simulink model "STOICAL_example_3_Step00_ExistingModell"  (R2014b)
settings: Solver=ode4  StartTime=0.0  StopTime=1  FixedStep=50E-6  RelTol=1e-3
model workspace (MAT data in the model file):
  STOVICAL.SignalSaveOptions.ReturnWorkspaceOutputs = 'on'
  STOVICAL.SignalSaveOptions.ReturnWorkspaceOutputsName = 'simout_obj'
  STOVICAL.SignalSaveOptions.SignalLogging = 'on'
  STOVICAL.SignalSaveOptions.SignalLoggingSaveFormat = 'Dataset'
  STOVICAL.SignalSaveOptions.SignalLoggingName = 'STOVICAL_LoggedSignals'
  STOVICAL.ParameterDefinition.BlkNameFull{1} = 'Step amplitude
    | #PARAM#Amplitude'
  STOVICAL.ParameterDefinition.BlkNameFull{2} = 'Dynamic System
    | #PARAM#w0#damp'
  STOVICAL.ParameterDefinition.BlkNameFull{3} = 'Static System
    | modelled
    | by gain block
    | #PARAM#SystemGain'
  STOVICAL.ParameterDefinition.BlkNameFull{4} = 'Dynamic System
    | #PARAM#w0#damp'
  STOVICAL.ParameterDefinition.BlkNameShort{1} = 'Step amplitude
    | '
  STOVICAL.ParameterDefinition.BlkNameShort{2} = 'Dynamic System
    | '
  STOVICAL.ParameterDefinition.BlkNameShort{3} = 'Static System
    | modelled
    | by gain block
    | '
  STOVICAL.ParameterDefinition.BlkNameShort{4} = 'Dynamic System
    | '
  STOVICAL.ParameterDefinition.BlkHandle = [8.0009765625; 15.0009765625; 21.0024414062; 15.0009765625]
  STOVICAL.ParameterDefinition.ParamName = {'Amplitude'; 'w0'; 'SystemGain'; 'damp'}
  STOVICAL.ParameterDefinition.BlkPath{1} = 'STOICAL_example_2_Step03_Activation/#UNIT#Stimulus/Step amplitude
    | #PARAM#Amplitude'
  STOVICAL.ParameterDefinition.BlkPath{2} = 'STOICAL_example_2_Step03_Activation/#UNIT#System/Dynamic System
    | #PARAM#w0#damp'
  STOVICAL.ParameterDefinition.BlkPath{3} = 'STOICAL_example_2_Step03_Activation/#UNIT#System/Static System
    | modelled
    | by gain block
    | #PARAM#SystemGain'
  STOVICAL.ParameterDefinition.BlkPath{4} = 'STOICAL_example_2_Step03_Activation/#UNIT#System/Dynamic System
    | #PARAM#w0#damp'
  STOVICAL.ParameterDefinition.BlkType = {'Constant'; 'SubSystem'; 'Gain'; 'SubSystem'}
  STOVICAL.ParameterDefinition.BlkMaskType = {''; ''; ''; ''}
  STOVICAL.ParameterDefinition.ParentalBlockPath = {'STOICAL_example_2_Step03_Activation/#UNIT#Stimulus'; 'STOICAL_example_2_Step03_Activation/#UNIT#System'; 'STOICAL_example_2_Step03_Activation/#UNIT#System'; 'STOICAL_example_2_Step03_Activation/#UNIT#System'}
  STOVICAL.ParameterDefinition.ParentalBlockHandle = [5.02294921875; 13.0029296875; 13.0029296875; 13.0029296875]
  STOVICAL.ParameterDefinition.Belongs2SubsystemHdl = [5.02294921875; 15.0009765625; 13.0029296875; 15.0009765625]
  STOVICAL.ParameterDefinition.NrParams = 4
  STOVICAL.ParameterDefinition.BlkField2Set = {'Value'; 'w0'; 'Gain'; 'damp'}
  STOVICAL.ParameterDefinition.BlkFieldSyntax = {'#'; '#'; '#'; '#'}
  STOVICAL.ParameterDefinition.ParamVariable = {'param_9ba35cf139ae8d049712606822772694'; 'param_518f5dd230dc6df197dc8805b8657145'; 'param_b7a2875e19f2aaba8a6b37e383b6fdf1'; 'param_13ac9ebe924e8dfd32ee0d3deb3cd2af'}
  STOVICAL.ParameterDefinition.LabelPath = {'#Stimulus#Amplitude'; '#System#w0'; '#System#SystemGain'; '#System#damp'}
  STOVICAL.ParameterDefinition.ParamDefaultValue = {'2'; '50'; '5'; '1/sqrt(2)'}
  STOVICAL.SignalDefinition.ParentalBlockPath = {'STOICAL_example_2_Step03_Activation'; 'STOICAL_example_2_Step03_Activation'}
  STOVICAL.SignalDefinition.ParentalBlockHandle = [3.0009765625; 3.0009765625]
  STOVICAL.SignalDefinition.NameInDiagram = {'#SIG#stimulus'; '#SIG#response'}
  STOVICAL.SignalDefinition.SourceBlockPath = {'STOICAL_example_2_Step03_Activation/#UNIT#Stimulus'; 'STOICAL_example_2_Step03_Activation/#UNIT#System'}
  STOVICAL.SignalDefinition.SourceBlockPort = [1; 1]
  STOVICAL.SignalDefinition.SourceBlockHandle = [5.02294921875; 13.0029296875]
  STOVICAL.SignalDefinition.Handle = [1948.00146484; 1949.01672363]
  STOVICAL.SignalDefinition.NrSig = 2
  STOVICAL.SignalDefinition.NameOfLogVar = {'logsig_643e3731b0c65fb38afb5e4f06d06a3f'; 'logsig_ee10c39bc06b89f4e4e488efcbc6167c'}
  STOVICAL.SignalDefinition.NameOfLogVarMode = {'Custom'; 'Custom'}
  STOVICAL.SignalDefinition.DoLog = [1; 1]
  STOVICAL.SignalDefinition.LabelPath = {'#stimulus'; '#response'}
  STOVICAL.VariantDefinition.NodeHandle = [3.0009765625; 5.02294921875; 13.0029296875; 15.0009765625]
  STOVICAL.VariantDefinition.NodeName{1} = 'STOICAL_example_2_Step03_Activation'
  STOVICAL.VariantDefinition.NodeName{2} = '#UNIT#Stimulus'
  STOVICAL.VariantDefinition.NodeName{3} = '#UNIT#System'
  STOVICAL.VariantDefinition.NodeName{4} = 'Dynamic System
    | #PARAM#w0#damp'
  STOVICAL.VariantDefinition.IsVariantSubsystem = [0; 0; 0; 0]
  STOVICAL.VariantDefinition.NodeLevel = [1; 2; 2; 3]
  STOVICAL.VariantDefinition.NodePath{1} = 'STOICAL_example_2_Step03_Activation'
  STOVICAL.VariantDefinition.NodePath{2} = 'STOICAL_example_2_Step03_Activation/#UNIT#Stimulus'
  STOVICAL.VariantDefinition.NodePath{3} = 'STOICAL_example_2_Step03_Activation/#UNIT#System'
  STOVICAL.VariantDefinition.NodePath{4} = 'STOICAL_example_2_Step03_Activation/#UNIT#System/Dynamic System
    | #PARAM#w0#damp'
  STOVICAL.VariantDefinition.IsVariant = [0; 0; 0; 0]
  STOVICAL.VariantDefinition.VSNodeIdxofVariant = [0; 0; 0; 0]
  STOVICAL.VariantDefinition.VSVariantsCount = [0; 0; 0; 0]
  STOVICAL.VariantDefinition.VSVariantsBlkHdls = {[]; []; []; []}
  STOVICAL.VariantDefinition.VSVariantsNodeIdx = {[]; []; []; []}
  STOVICAL.VariantDefinition.VSControlVariable = {[]; []; []; []}
  STOVICAL.VariantDefinition.VSVariantHasNr = [0; 0; 0; 0]
  STOVICAL.VariantDefinition.LabelPath = {[]; []; []; []}
  param_ec6e274da2c23e664dfdc874ac252818 = '2'
  param_afc1e04cc1c158b687408e5b6ea19d06 = '5'
  param_9ba35cf139ae8d049712606822772694 = '2'
  param_518f5dd230dc6df197dc8805b8657145 = '50'
  param_b7a2875e19f2aaba8a6b37e383b6fdf1 = '5'
  param_13ac9ebe924e8dfd32ee0d3deb3cd2af = '1/sqrt(2)'
settings Model: Creator=Wippenbeck  LastModifiedBy=Wippenbeck
settings DataIOCC: ReturnWorkspaceOutputs=on  SignalLoggingName=STOVICAL_LoggedSignals  ReturnWorkspaceOutputsName=simout_obj

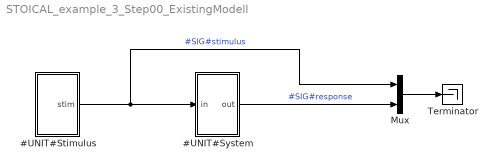
== system STOICAL_example_3_Step00_ExistingModell ==
  #UNIT#Stimulus : Subsystem
  #UNIT#System : Subsystem
  Mux : Mux  Inputs=2
  Terminator : Terminator
  wires:
  Mux/1 -> Terminator/1
  #UNIT#Stimulus/1(stim) -> #UNIT#System/1(in), Mux/1  "#SIG#stimulus"
  #UNIT#System/1(out) -> Mux/2  "#SIG#response"

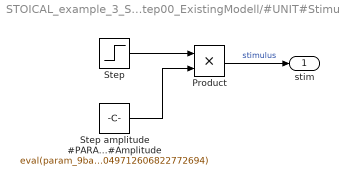
== system STOICAL_example_3_Step00_ExistingModell/#UNIT#Stimulus ==
  Product : Product
  Step : Step  Time=0.1  SampleTime=0
  Step amplitude #PARAM#Amplitude : Constant  Value=eval(param_9ba35cf139ae8d049712606822772694)
  stim : Outport
  wires:
  Step amplitude #PARAM#Amplitude/1 -> Product/2
  Product/1 -> stim/1  "stimulus"
  Step/1 -> Product/1

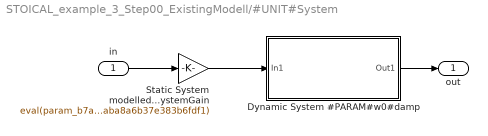
== system STOICAL_example_3_Step00_ExistingModell/#UNIT#System ==
  in : Inport
  Dynamic System #PARAM#w0#damp : Subsystem  mask{w0=eval(param_518f5dd230dc6df197dc8805b8657145), damp=eval(param_13ac9ebe924e8dfd32ee0d3deb3cd2af)}
      mask prompts: w0 "Natural frequency w0 [rad/s]"; damp "Damping zeta [1]"
      mask help:
      | Dynamical system of the form
      |
      | G(s) = w0^2 / (s^2 + 2*zeta*w0*s + wo^2)
  Static System modelled by gain block #PARAM#SystemGain : Gain  Gain=eval(param_b7a2875e19f2aaba8a6b37e383b6fdf1)
  out : Outport
  wires:
  in/1 -> Static System modelled by gain block #PARAM#SystemGain/1
  Static System modelled by gain block #PARAM#SystemGain/1 -> Dynamic System #PARAM#w0#damp/1(In1)
  Dynamic System #PARAM#w0#damp/1(Out1) -> out/1

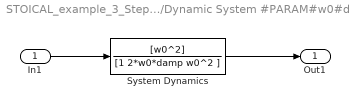
== system STOICAL_example_3_Step00_ExistingModell/#UNIT#System/Dynamic System #PARAM#w0#damp ==
  In1 : Inport
  System Dynamics : TransferFcn  Numerator=[w0^2]  Denominator=[1 2*w0*damp w0^2 ]
  Out1 : Outport
  wires:
  System Dynamics/1 -> Out1/1
  In1/1 -> System Dynamics/1
